simulink model "Full_model"  (R2020a)
settings: Solver=VariableStepAuto  StartTime=0.0  StopTime=inf  RelTol=1e-3
model workspace (MAT data in the model file):
  WinSize = Simulink.Parameter
  WinSize.Value = 16
  WinSize.DataType = 'double'
  WinSize.Dimensions = [1 1]
  fc_bandpass = Simulink.Parameter
  fc_bandpass.Value = [0.05 0.26]
  fc_bandpass.DataType = 'double'
  fc_bandpass.Dimensions = [1 2]
undefined symbols (not defined in the file or in its folder): A1, A30722, A91496, C1, currentCFG_Cognata_Amp_Tobi_split_UB, I1, J30722, P91496, UB, W1, W91496
libraries: gtecHighspeedLib x13, robotlib x6, dspnetwork x1, gUSBamplib x1, TobiiEyeTrackerLib x1
settings Model: Creator=LAB-OREN3  LastModifiedBy=LAB-OREN3

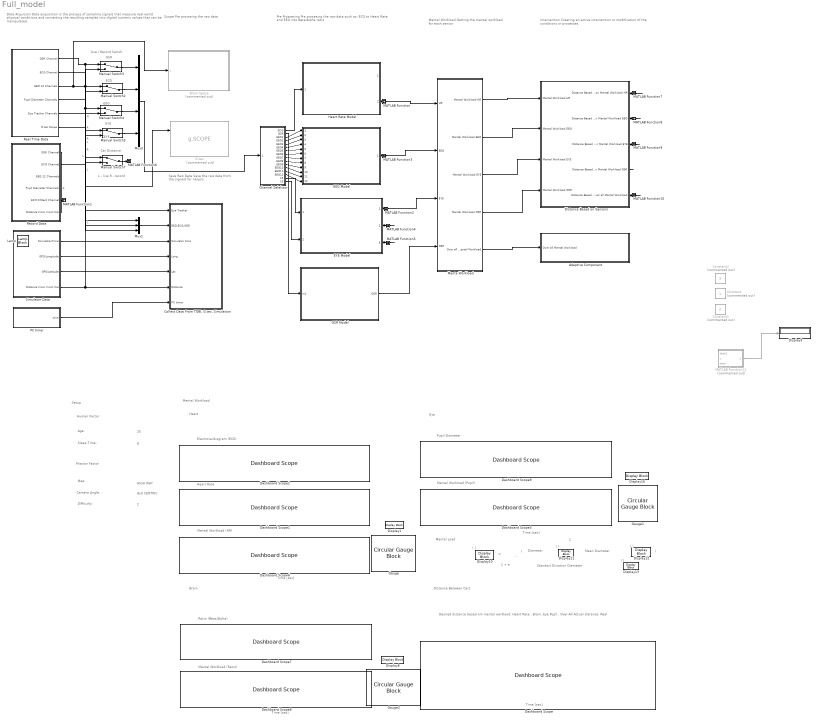
== system Full_model ==
  note: L - live
      | R - record
  note: Live / Record Switch
  note: GSR
  note: Intervention
      | Creating an active intervention or modification of the conditions or processes
  note: Save Raw Data
      | Save the raw data from the signals for nalysis
  note: Mental Workload
      | Getting the mental workload for each sensor
  note: Pre Prossesing
      | Pre prosseing the raw data such as:
      | ECG to Heart Rate and EEG into Beta/Alpha ratio
  note: Data Acquision
      | Data acquisition is the process of sampling signals that measure real-world physical conditions and converting the resulting samples into digital numeric values that can be manipulated.
  note: Time [sec]
  note: Electrocardiogram (ECG)
  note: . Distance Between Cars
  note: Mean Diameter
  note: 25
  note: Human Factor
  note: Standart Diviation Diameter
  note: Age:
  note: HIGH WAY
  note: Difficulty:
  note: Mental Workload (Pupil)
  note: ( )
  note: 8
  note: 1 + e
  note: Camera Angle: :
  note: Heart Rate
  note: Time [sec]
  note: Brain
  note: ( )
  note: Pupil Diameter
  note: . Setup
  note: 2
  note: ( )
  note: 1
  note: Desired distance based om mental worklaod:
      | Heart Rate , Brain, Eye Pupil , Over-All
      |
      | Actual distance: Real
  note: (
  note: Mission Factor
  note: Ratio (Beta/Alpha)
  note: -
  note: Mental Workload (HR)
  note: Sleep Time:
  note: ( )
  note: Diameter
  note: Mental Load
  note: )
  note: =
  note: Time [sec]
  note: Eye
  note: Mental Workload (Ratio)
  note: Time [sec]
  note: Mental Workload
  note: Heart
  note: Map:
  note: ALO CENTRIC
  note: ECG
  note: EEG
  note: EYE
  note: Car Distance
  note: EYE
  note: Scope
      | Pre prosseing the raw data
  Adaptive Component : Subsystem
  Brain Space : Subsystem  Commented=on
  Channel Selelctor : Subsystem
  "Collect Data From TOBI, G.tec, Simulation" : Subsystem
  Constant : Constant  Commented=on  SampleTime=0.5
  Constant1 : Constant  Commented=on  Value=2  SampleTime=0.5
  Constant2 : Constant  Commented=on  Value=3  SampleTime=0.5
  Dashboard Scope : DashboardScope  ShowInitialText=off  TimeSpan=10  Ymin=-1  Ymax=20  LegendPosition=Hide  ScaleAtStop=off
  Dashboard Scope1 : DashboardScope  TimeSpan=10  Ymin=0  Ymax=100  LegendPosition=Hide  ScaleAtStop=off
  Dashboard Scope2 : DashboardScope  TimeSpan=10  Ymin=-3000  Ymax=1000  LegendPosition=Hide  ScaleAtStop=off
  Dashboard Scope3 : DashboardScope  TimeSpan=10  Ymin=0  Ymax=1  LegendPosition=Hide  ScaleAtStop=off
  Dashboard Scope6 : DashboardScope  TimeSpan=10  Ymin=0  Ymax=1  LegendPosition=Hide  ScaleAtStop=off
  Dashboard Scope7 : DashboardScope  TimeSpan=10  Ymin=0  Ymax=0.5  LegendPosition=Hide  ScaleAtStop=off
  Dashboard Scope8 : DashboardScope  TimeSpan=10  Ymin=0  Ymax=1  LegendPosition=Hide  ScaleAtStop=off
  Dashboard Scope9 : DashboardScope  TimeSpan=10  Ymin=0  Ymax=5  LegendPosition=Hide  ScaleAtStop=off
  Display{1,8,10..11,13,16} (6 alike) : DisplayBlock  LabelPosition=Hide  Format=bank  Transparency=1
  Display12 : DisplayBlock  LabelPosition=Hide  Format=bank  Transparency=1  Layout=Fill available space
  Display3 : Display
  Distance Based on Sensors : Subsystem
  EEG Model : Subsystem  ReferencedSubsystem=EEG_Ratio_Model
  EYE Model : Subsystem  ReferencedSubsystem=Pupil_Diameter_Model
  G.tec : gtecHighspeedLib/g.SCOPE  Commented=on
      settings: SourceProductName=g.HIsys Library
  GSR Model : Subsystem
  Gauge : CircularGaugeBlock  LabelPosition=Hide  ScaleMax=1  TickInterval=0.2
  Gauge1 : CircularGaugeBlock  LabelPosition=Hide  ScaleMax=1  TickInterval=0.2
  Gauge2 : CircularGaugeBlock  LabelPosition=Hide  ScaleMax=1  TickInterval=0.2
  Heart Rate Model : Subsystem  ReferencedSubsystem=Heart_Rate_Model
  Lamp : LampBlock  LabelPosition=Hide
  MATLAB Function : MATLAB Function  TreatAsAtomicUnit=on
  MATLAB Function1 : MATLAB Function  TreatAsAtomicUnit=on
  MATLAB Function10 : MATLAB Function  TreatAsAtomicUnit=on
  MATLAB Function11 : MATLAB Function  Commented=on  TreatAsAtomicUnit=on
  MATLAB Function2 : MATLAB Function  TreatAsAtomicUnit=on
  MATLAB Function3 : MATLAB Function  TreatAsAtomicUnit=on
  MATLAB Function4 : MATLAB Function  TreatAsAtomicUnit=on
  MATLAB Function5 : MATLAB Function  TreatAsAtomicUnit=on
  MATLAB Function6 : MATLAB Function  TreatAsAtomicUnit=on
  MATLAB Function7 : MATLAB Function  TreatAsAtomicUnit=on
  MATLAB Function8 : MATLAB Function  TreatAsAtomicUnit=on
  MATLAB Function9 : MATLAB Function  TreatAsAtomicUnit=on
  Manual Switch{2..5,7} (5 alike) : ManualSwitch
  "Menta Workload " : Subsystem
  Mux1 : Mux  Inputs=3
  Mux3 : Mux
  PC timer : Subsystem
  Real Time Data : Subsystem
  Record Data : Subsystem
  Simulator Data : Subsystem
  wires:
  Simulator Data/2(GPS/Longitude) -> "Collect Data From TOBI, G.tec, Simulation"/4(Long)
  Simulator Data/3(GPS/Latitude) -> "Collect Data From TOBI, G.tec, Simulation"/5(Lat)
  Simulator Data/1(SimulationTime) -> "Collect Data From TOBI, G.tec, Simulation"/3(Simulator time)
  Simulator Data/4(Distance From Front Car) -> Manual Switch7/1, "Collect Data From TOBI, G.tec, Simulation"/6(Distance)  "L"
  Heart Rate Model/2 -> MATLAB Function/1(u)
  EYE Model/1 -> MATLAB Function2/1(u)
  GSR Model/1(GSR) -> "Menta Workload "/4(GSR)
  "Menta Workload "/2(Mental Workload EEG) -> Distance Based on Sensors/2(Mental Workload EEG)
  "Menta Workload "/5("Over all Mental Workload ") -> Adaptive Component/1("Over all Mental Workload ")
  Distance Based on Sensors/1(Distance Based on Mental Workload HR) -> MATLAB Function7/1(u)
  Distance Based on Sensors/2(Distance Based on Mental Workload EEG) -> MATLAB Function8/1(u)
  Distance Based on Sensors/3(Distance Based on Mental Workload EYE) -> MATLAB Function9/1(u)
  Distance Based on Sensors/4(Distance Based on Mental Workload GSR) -> ?
  Distance Based on Sensors/5(Distance Based on Over all Mental Workload) -> MATLAB Function10/1(u)
  EYE Model/2 -> MATLAB Function4/1(u)
  EYE Model/3 -> MATLAB Function5/1(u)
  Channel Selelctor/2(GSR) -> GSR Model/1(In1)
  Channel Selelctor/1(ECG) -> Heart Rate Model/1
  Channel Selelctor/3(EEG1) -> EEG Model/1
  Channel Selelctor/4(EEG2) -> EEG Model/2
  Channel Selelctor/5(EEG3) -> EEG Model/3
  Channel Selelctor/6(EEG4) -> EEG Model/4
  Channel Selelctor/7(EEG5) -> EEG Model/5
  Channel Selelctor/8(EEG6) -> EEG Model/6
  Channel Selelctor/9(EEG7) -> EEG Model/7
  Channel Selelctor/10(EEG8) -> EEG Model/8
  Channel Selelctor/11(EEG9) -> EEG Model/9
  Channel Selelctor/12(EEG10) -> EEG Model/10
  Channel Selelctor/13(EEG11) -> EEG Model/11
  Channel Selelctor/14(EEG12) -> EEG Model/12
  Channel Selelctor/15(Pupil right) -> EYE Model/1
  Channel Selelctor/16(Pupil Left) -> EYE Model/2
  Manual Switch3/1 -> Mux3/1
  Manual Switch2/1 -> Mux3/2
  Manual Switch4/1 -> Mux3/3
  Manual Switch5/1 -> Mux3/4
  Record Data/1(GSR Channel) -> Manual Switch3/2  "R"
  Real Time Data/1(GSR Channel) -> Manual Switch3/1, Mux1/1  "L"
  Real Time Data/2(ECG Channel) -> Mux1/2, Manual Switch2/1  "L"
  Record Data/2(ECG Channel) -> Manual Switch2/2  "R"
  Record Data/3(EEG 12 Channels) -> Manual Switch4/2  "R"
  Real Time Data/3(EEG 12 Channels) -> Mux1/3, Manual Switch4/1, Brain Space/1(L)  "L"
  Record Data/4(" Pupil Diameter Channels ") -> Manual Switch5/2  "R"
  Manual Switch7/1 -> MATLAB Function6/1(u)
  Record Data/5(ECG Filtterd Channel) -> MATLAB Function1/1(u)
  Real Time Data/5(Eye Tracker Channels) -> "Collect Data From TOBI, G.tec, Simulation"/1(Eye Tracker)
  Mux3/1 -> Channel Selelctor/1(16x1 vec)
  Mux1/1 -> "Collect Data From TOBI, G.tec, Simulation"/2("EEG,ECG,GSR ")
  Record Data/6(Distance From Front Car) -> Manual Switch7/2  "R"
  PC timer/1(time) -> "Collect Data From TOBI, G.tec, Simulation"/7(PC timer)
  Real Time Data/4(Pupil Diameter Channels) -> Manual Switch5/1
  MATLAB Function/1(y) -> "Menta Workload "/1(HR)
  MATLAB Function2/1(y) -> "Menta Workload "/3(EYE)
  EEG Model/1 -> MATLAB Function3/1(u)
  MATLAB Function3/1(y) -> "Menta Workload "/2(EEG)
  MATLAB Function4/1(y) -> ?
  MATLAB Function5/1(y) -> ?
  MATLAB Function7/1(y) -> ?
  MATLAB Function8/1(y) -> ?
  MATLAB Function9/1(y) -> ?
  MATLAB Function10/1(y) -> ?
  "Menta Workload "/3(Mental Workload EYE) -> Distance Based on Sensors/3(Mental Workload EYE)
  MATLAB Function11/1(y) -> Display3/1
  "Menta Workload "/1(Mental Workload HR) -> Distance Based on Sensors/1(Mental Workload HR)
  "Menta Workload "/4(Mental Workload GSR) -> Distance Based on Sensors/4(Mental Workload GSR)
  Real Time Data/6(G.tec Scope) -> G.tec/1

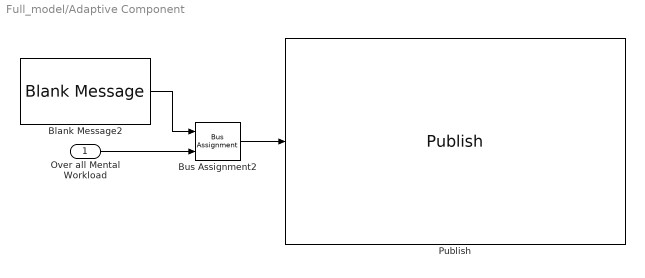
== system Full_model/Adaptive Component ==
  "Over all Mental Workload " : Inport
  Blank Message2 : robotlib/Blank Message  messageClass=Message  entityType=std_msgs/Float64  messageType=std_msgs/Float64  SampleTime=0
  Bus Assignment2 : BusAssignment  AssignedSignals=Data
  Publish : robotlib/Publish  topicSource=Specify your own  topic=/HR  messageType=std_msgs/Float64  messageQueueLength=1
  wires:
  "Over all Mental Workload "/1 -> Bus Assignment2/2
  Blank Message2/1 -> Bus Assignment2/1
  Bus Assignment2/1 -> Publish/1

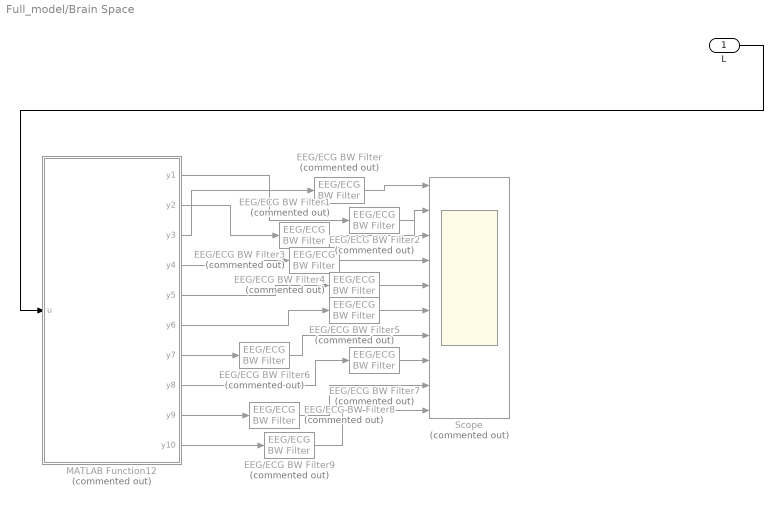
== system Full_model/Brain Space ==
  L : Inport
  EEG/ECG BW Filter{,1..9} (10 alike) : gtecHighspeedLib/EEG//ECG BW Filter  Commented=on  Order=6  LowerFreq=0.1  UpperFreq=30  SampFreq=512
      settings: SourceProductName=g.HIsys Library
  MATLAB Function12 : MATLAB Function  Commented=on  TreatAsAtomicUnit=on
  Scope : Scope  Commented=on  NumInputPorts=10
  wires:
  MATLAB Function12/1(y1) -> EEG/ECG BW Filter2/1
  MATLAB Function12/10(y10) -> EEG/ECG BW Filter9/1
  MATLAB Function12/4(y4) -> EEG/ECG BW Filter3/1
  MATLAB Function12/6(y6) -> EEG/ECG BW Filter5/1
  EEG/ECG BW Filter8/1 -> Scope/9
  EEG/ECG BW Filter3/1 -> Scope/4
  MATLAB Function12/2(y2) -> EEG/ECG BW Filter1/1
  EEG/ECG BW Filter5/1 -> Scope/6
  EEG/ECG BW Filter4/1 -> Scope/5
  EEG/ECG BW Filter7/1 -> Scope/8
  EEG/ECG BW Filter/1 -> Scope/1
  L/1 -> MATLAB Function12/1(u)
  MATLAB Function12/7(y7) -> EEG/ECG BW Filter6/1
  MATLAB Function12/8(y8) -> EEG/ECG BW Filter7/1
  EEG/ECG BW Filter1/1 -> Scope/2
  MATLAB Function12/9(y9) -> EEG/ECG BW Filter8/1
  MATLAB Function12/5(y5) -> EEG/ECG BW Filter4/1
  EEG/ECG BW Filter9/1 -> Scope/10
  EEG/ECG BW Filter2/1 -> Scope/3
  EEG/ECG BW Filter6/1 -> Scope/7
  MATLAB Function12/3(y3) -> EEG/ECG BW Filter/1

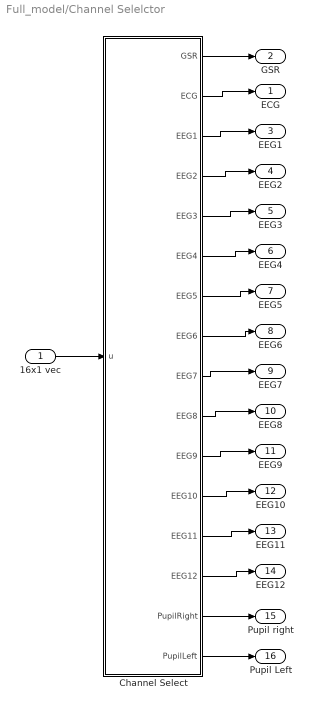
== system Full_model/Channel Selelctor ==
  16x1 vec : Inport
  " Channel Select" : MATLAB Function  TreatAsAtomicUnit=on
  ECG : Outport
  GSR : Outport  Port=2
  EEG1 : Outport  Port=3
  EEG2 : Outport  Port=4
  EEG3 : Outport  Port=5
  EEG4 : Outport  Port=6
  EEG5 : Outport  Port=7
  EEG6 : Outport  Port=8
  EEG7 : Outport  Port=9
  EEG8 : Outport  Port=10
  EEG9 : Outport  Port=11
  EEG10 : Outport  Port=12
  EEG11 : Outport  Port=13
  EEG12 : Outport  Port=14
  Pupil right : Outport  Port=15
  Pupil Left : Outport  Port=16
  wires:
  16x1 vec/1 -> " Channel Select"/1(u)
  " Channel Select"/1(GSR) -> GSR/1
  " Channel Select"/2(ECG) -> ECG/1
  " Channel Select"/3(EEG1) -> EEG1/1
  " Channel Select"/4(EEG2) -> EEG2/1
  " Channel Select"/5(EEG3) -> EEG3/1
  " Channel Select"/6(EEG4) -> EEG4/1
  " Channel Select"/7(EEG5) -> EEG5/1
  " Channel Select"/8(EEG6) -> EEG6/1
  " Channel Select"/9(EEG7) -> EEG7/1
  " Channel Select"/10(EEG8) -> EEG8/1
  " Channel Select"/11(EEG9) -> EEG9/1
  " Channel Select"/12(EEG10) -> EEG10/1
  " Channel Select"/13(EEG11) -> EEG11/1
  " Channel Select"/14(EEG12) -> EEG12/1
  " Channel Select"/15(PupilRight) -> Pupil right/1
  " Channel Select"/16(PupilLeft) -> Pupil Left/1

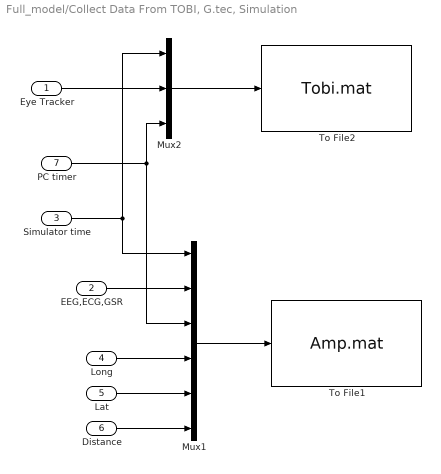
== system Full_model/Collect Data From TOBI, G.tec, Simulation ==
  Eye Tracker : Inport
  "EEG,ECG,GSR " : Inport  Port=2
  Simulator time : Inport  Port=3
  Long : Inport  Port=4
  Lat : Inport  Port=5
  Distance : Inport  Port=6
  PC timer : Inport  Port=7
  Mux1 : Mux  Inputs=6
  Mux2 : Mux  Inputs=3
  To File1 : ToFile  Filename=Amp.mat  MatrixName=Ampdata
  To File2 : ToFile  Filename=Tobi.mat  MatrixName=Tobidata
  wires:
  Eye Tracker/1 -> Mux2/2
  Simulator time/1 -> Mux1/1, Mux2/1
  Mux1/1 -> To File1/1
  Mux2/1 -> To File2/1
  Long/1 -> Mux1/4
  Distance/1 -> Mux1/6
  "EEG,ECG,GSR "/1 -> Mux1/2
  Lat/1 -> Mux1/5
  PC timer/1 -> Mux1/3, Mux2/3

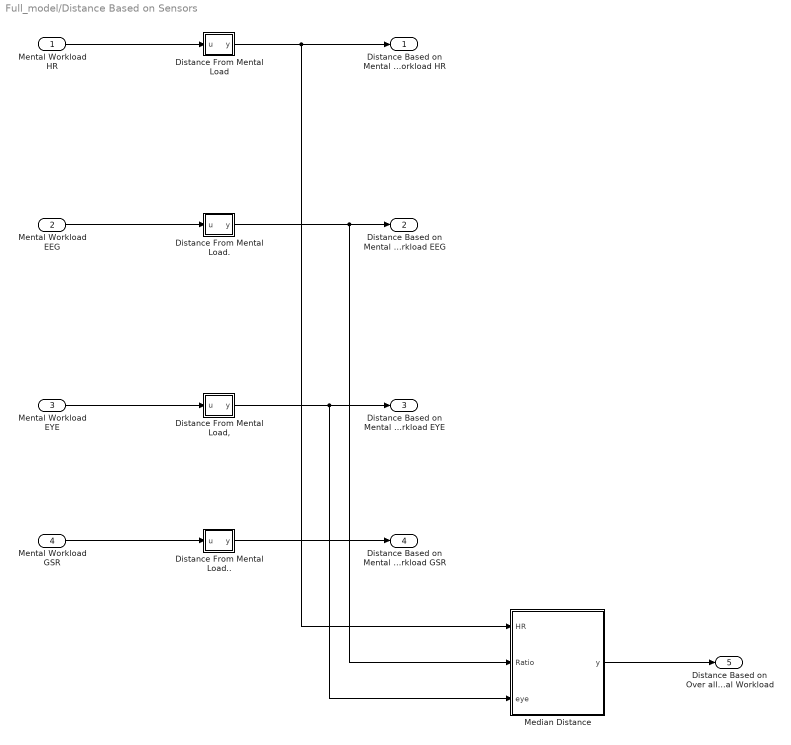
== system Full_model/Distance Based on Sensors ==
  Mental Workload HR : Inport
  Mental Workload EEG : Inport  Port=2
  Mental Workload EYE : Inport  Port=3
  Mental Workload GSR : Inport  Port=4
  Distance From Mental Load : MATLAB Function  TreatAsAtomicUnit=on
  Distance From Mental Load, : MATLAB Function  TreatAsAtomicUnit=on
  Distance From Mental Load. : MATLAB Function  TreatAsAtomicUnit=on
  Distance From Mental Load.. : MATLAB Function  TreatAsAtomicUnit=on
  Median Distance : MATLAB Function  TreatAsAtomicUnit=on
  Distance Based on Mental Workload HR : Outport
  Distance Based on Mental Workload EEG : Outport  Port=2
  Distance Based on Mental Workload EYE : Outport  Port=3
  Distance Based on Mental Workload GSR : Outport  Port=4
  Distance Based on Over all Mental Workload : Outport  Port=5
  wires:
  Distance From Mental Load,/1(y) -> Distance Based on Mental Workload EYE/1, Median Distance/3(eye)
  Mental Workload HR/1 -> Distance From Mental Load/1(u)
  Distance From Mental Load../1(y) -> Distance Based on Mental Workload GSR/1
  Mental Workload EEG/1 -> Distance From Mental Load./1(u)
  Mental Workload GSR/1 -> Distance From Mental Load../1(u)
  Distance From Mental Load/1(y) -> Distance Based on Mental Workload HR/1, Median Distance/1(HR)
  Mental Workload EYE/1 -> Distance From Mental Load,/1(u)
  Distance From Mental Load./1(y) -> Distance Based on Mental Workload EEG/1, Median Distance/2(Ratio)
  Median Distance/1(y) -> Distance Based on Over all Mental Workload/1

== system Full_model/GSR Model ==
  In1 : Inport
  GSR : Outport
  wires:
  In1/1 -> GSR/1

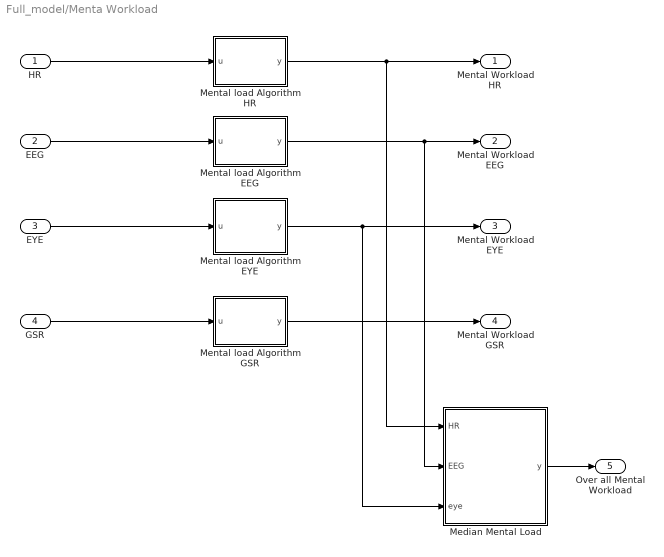
== system Full_model/Menta Workload  ==
  HR : Inport
  EEG : Inport  Port=2
  EYE : Inport  Port=3
  GSR : Inport  Port=4
  Median Mental Load : MATLAB Function  TreatAsAtomicUnit=on
  Mental load Algorithm EEG : MATLAB Function  TreatAsAtomicUnit=on
  Mental load Algorithm EYE : MATLAB Function  TreatAsAtomicUnit=on
  Mental load Algorithm GSR : MATLAB Function  TreatAsAtomicUnit=on
  Mental load Algorithm HR : MATLAB Function  TreatAsAtomicUnit=on
  Mental Workload HR : Outport
  Mental Workload EEG : Outport  Port=2
  Mental Workload EYE : Outport  Port=3
  Mental Workload GSR : Outport  Port=4
  "Over all Mental Workload " : Outport  Port=5
  wires:
  HR/1 -> Mental load Algorithm HR/1(u)
  Mental load Algorithm HR/1(y) -> Mental Workload HR/1, Median Mental Load/1(HR)
  EEG/1 -> Mental load Algorithm EEG/1(u)
  Mental load Algorithm EEG/1(y) -> Median Mental Load/2(EEG), Mental Workload EEG/1
  EYE/1 -> Mental load Algorithm EYE/1(u)
  Mental load Algorithm EYE/1(y) -> Mental Workload EYE/1, Median Mental Load/3(eye)
  GSR/1 -> Mental load Algorithm GSR/1(u)
  Mental load Algorithm GSR/1(y) -> Mental Workload GSR/1
  Median Mental Load/1(y) -> "Over all Mental Workload "/1

== system Full_model/PC timer ==
  PC timer : MATLAB Function  TreatAsAtomicUnit=on
  time : Outport
  wires:
  PC timer/1(z) -> time/1

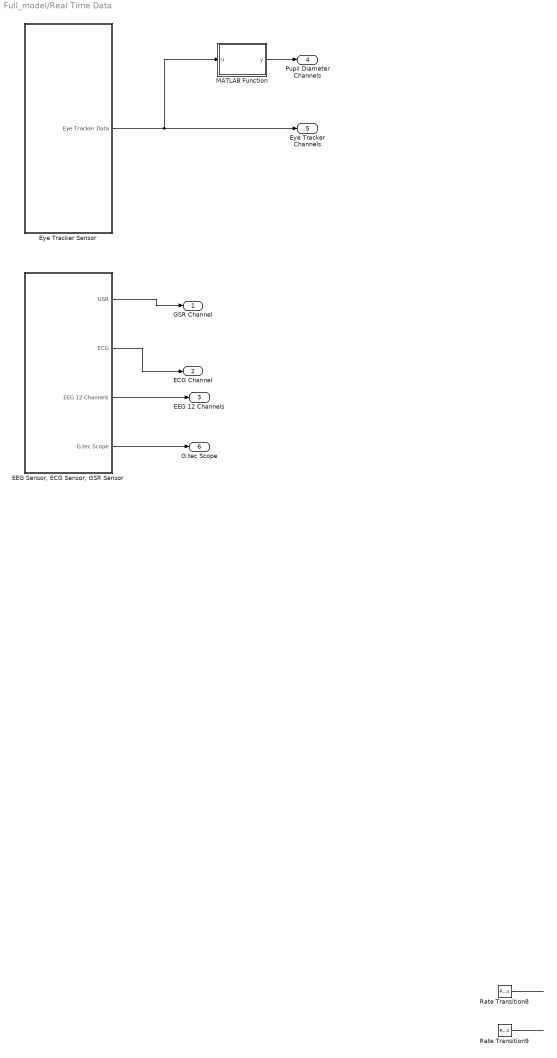
== system Full_model/Real Time Data ==
  "EEG Sensor, ECG Sensor, GSR Sensor " : Subsystem
  Eye Tracker Sensor : Subsystem
  MATLAB Function : MATLAB Function  TreatAsAtomicUnit=on
  Rate Transition8 : RateTransition  Deterministic=off  OutPortSampleTimeOpt=Inherit
  Rate Transition9 : RateTransition  Deterministic=off  OutPortSampleTimeOpt=Inherit
  GSR Channel : Outport
  ECG Channel : Outport  Port=2
  EEG 12 Channels : Outport  Port=3
  Pupil Diameter Channels : Outport  Port=4
  Eye Tracker Channels : Outport  Port=5
  G.tec Scope : Outport  Port=6
  wires:
  Eye Tracker Sensor/1(Eye Tracker Data) -> MATLAB Function/1(u), Eye Tracker Channels/1
  Rate Transition8/1 -> ?
  Rate Transition9/1 -> ?
  "EEG Sensor, ECG Sensor, GSR Sensor "/1(GSR) -> GSR Channel/1
  "EEG Sensor, ECG Sensor, GSR Sensor "/2(ECG) -> ECG Channel/1
  "EEG Sensor, ECG Sensor, GSR Sensor "/3(EEG 12 Channels) -> EEG 12 Channels/1
  MATLAB Function/1(y) -> Pupil Diameter Channels/1
  "EEG Sensor, ECG Sensor, GSR Sensor "/4(G.tec Scope) -> G.tec Scope/1

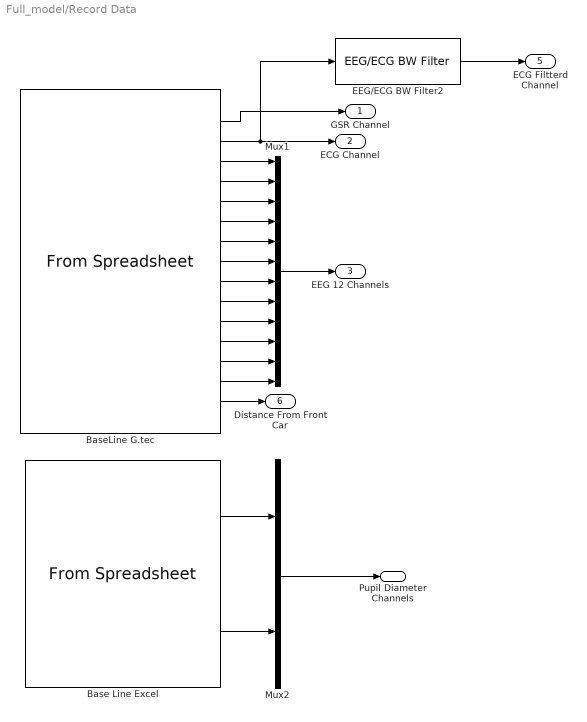
== system Full_model/Record Data ==
  Base Line Excel : FromSpreadsheet  FileName=C:\Users\LAB-OREN3\Desktop\CognataData\Participants_DATA\Test\3\Tobii Data of A3_458493_COMBINED_CAR_DELAY_50_TTC_15 at (18_15_7).xlsx  SheetName=גיליון1  Range=A1:A30722,I1:J30722  SampleTime=0.001953125
  BaseLine G.tec : FromSpreadsheet  FileName=C:\Users\LAB-OREN3\Desktop\CognataData\Participants_DATA\Test\1\g.techAmp Data of A6_473257_COMBINED_CUBE_DELAY_150_TTC_ML at (13;32;25).xlsx  SheetName=גיליון1  Range=A1:A91496,C1:P91496,W1:W91496  SampleTime=0.001953125
  EEG/ECG BW Filter2 : gtecHighspeedLib/EEG//ECG BW Filter  Order=6  LowerFreq=0.1  UpperFreq=30  SampFreq=512
      settings: SourceProductName=g.HIsys Library
  Mux1 : Mux  Inputs=12
  Mux2 : Mux  Inputs=2
  GSR Channel : Outport
  ECG Channel : Outport  Port=2
  EEG 12 Channels : Outport  Port=3
  " Pupil Diameter Channels " : Outport  Port=4
  ECG Filtterd Channel : Outport  Port=5
  Distance From Front Car : Outport  Port=6
  wires:
  BaseLine G.tec/5 -> Mux1/3
  BaseLine G.tec/13 -> Mux1/11
  BaseLine G.tec/10 -> Mux1/8
  BaseLine G.tec/11 -> Mux1/9
  BaseLine G.tec/14 -> Mux1/12
  BaseLine G.tec/12 -> Mux1/10
  BaseLine G.tec/8 -> Mux1/6
  BaseLine G.tec/4 -> Mux1/2
  BaseLine G.tec/9 -> Mux1/7
  BaseLine G.tec/6 -> Mux1/4
  BaseLine G.tec/7 -> Mux1/5
  BaseLine G.tec/3 -> Mux1/1
  BaseLine G.tec/15 -> Distance From Front Car/1
  BaseLine G.tec/2 -> ECG Channel/1, EEG/ECG BW Filter2/1
  BaseLine G.tec/1 -> GSR Channel/1
  Base Line Excel/2 -> Mux2/2
  Base Line Excel/1 -> Mux2/1
  Mux2/1 -> " Pupil Diameter Channels "/1
  EEG/ECG BW Filter2/1 -> ECG Filtterd Channel/1
  Mux1/1 -> EEG 12 Channels/1

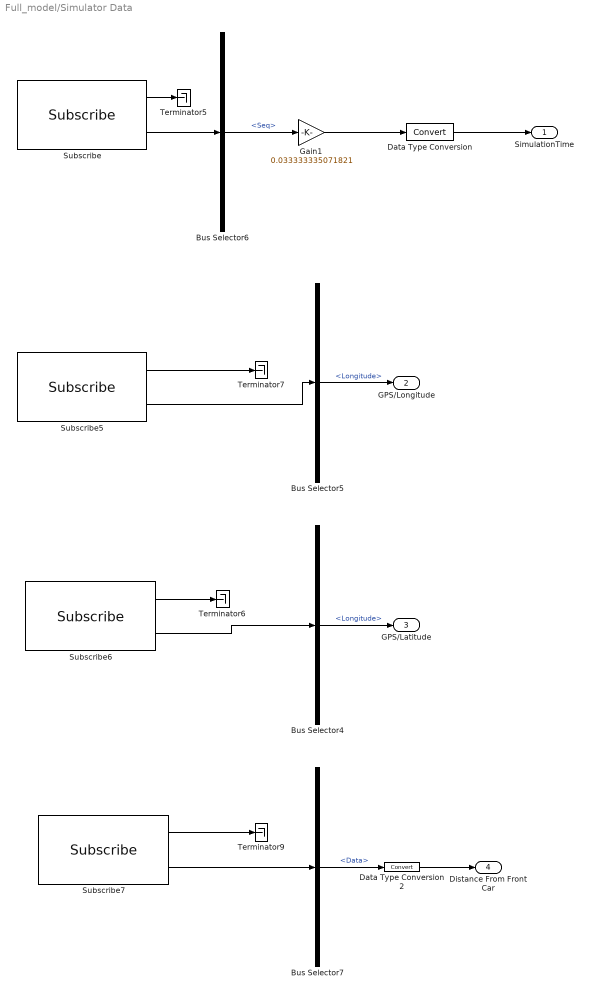
== system Full_model/Simulator Data ==
  Bus Selector4 : BusSelector  OutputSignals=Longitude
  Bus Selector5 : BusSelector  OutputSignals=Longitude
  Bus Selector6 : BusSelector  OutputSignals=Header.Seq
  Bus Selector7 : BusSelector  OutputSignals=Data
  Data Type Conversion : DataTypeConversion
  Data Type Conversion2 : DataTypeConversion
  Gain1 : Gain  Gain=0.033333335071821
  Subscribe : robotlib/Subscribe  topicSource=Specify your own  topic=/cognataSDK/GPS/info  messageType=sensor_msgs/NavSatFix  sampleTime=0.5  messageQueueLength=1
  Subscribe5 : robotlib/Subscribe  topicSource=Specify your own  topic=/cognataSDK/GPS/info  messageType=sensor_msgs/NavSatFix  sampleTime=-1  messageQueueLength=1
  Subscribe6 : robotlib/Subscribe  topicSource=Specify your own  topic=/cognataSDK/GPS/info  messageType=sensor_msgs/NavSatFix  sampleTime=-1  messageQueueLength=1
  Subscribe7 : robotlib/Subscribe  topicSource=Specify your own  topic=/Distance_topic  messageType=std_msgs/Float32  sampleTime=0.5  messageQueueLength=1
  Terminator{5..7,9} (4 alike) : Terminator
  SimulationTime : Outport
  GPS/Longitude : Outport  Port=2
  GPS/Latitude : Outport  Port=3
  Distance From Front Car : Outport  Port=4
  wires:
  Subscribe/1 -> Terminator5/1
  Bus Selector4/1 -> GPS/Latitude/1  "<Longitude>"
  Subscribe6/2 -> Bus Selector4/1
  Subscribe6/1 -> Terminator6/1
  Bus Selector5/1 -> GPS/Longitude/1  "<Longitude>"
  Subscribe5/2 -> Bus Selector5/1
  Subscribe5/1 -> Terminator7/1
  Subscribe/2 -> Bus Selector6/1
  Bus Selector6/1 -> Gain1/1  "<Seq>"
  Subscribe7/2 -> Bus Selector7/1
  Subscribe7/1 -> Terminator9/1
  Bus Selector7/1 -> Data Type Conversion2/1  "<Data>"
  Gain1/1 -> Data Type Conversion/1
  Data Type Conversion/1 -> SimulationTime/1
  Data Type Conversion2/1 -> Distance From Front Car/1

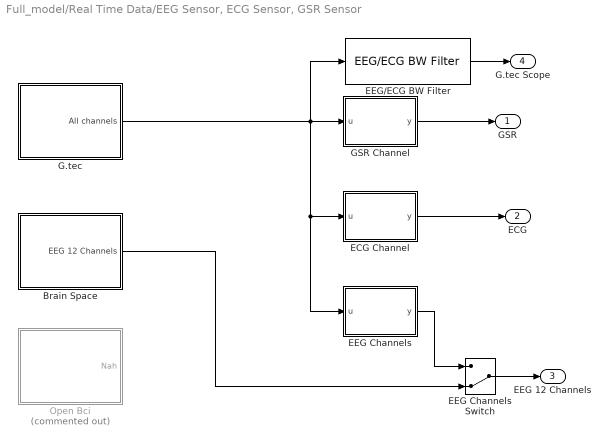
== system Full_model/Real Time Data/EEG Sensor, ECG Sensor, GSR Sensor  ==
  Brain Space : Subsystem
  "ECG Channel " : MATLAB Function  TreatAsAtomicUnit=on
  "EEG Channels " : MATLAB Function  TreatAsAtomicUnit=on
  EEG Channels Switch : ManualSwitch  CurrentSetting=0
  EEG/ECG BW Filter : gtecHighspeedLib/EEG//ECG BW Filter  Order=6  LowerFreq=0.1  UpperFreq=30  SampFreq=512
      settings: SourceProductName=g.HIsys Library
  G.tec : Subsystem
  GSR Channel : MATLAB Function  TreatAsAtomicUnit=on
  Open Bci : Subsystem  Commented=on
  GSR : Outport
  ECG : Outport  Port=2
  EEG 12 Channels : Outport  Port=3
  G.tec Scope : Outport  Port=4
  wires:
  G.tec/1(All channels) -> "EEG Channels "/1(u), "ECG Channel "/1(u), GSR Channel/1(u), EEG/ECG BW Filter/1
  GSR Channel/1(y) -> GSR/1
  "ECG Channel "/1(y) -> ECG/1
  "EEG Channels "/1(y) -> EEG Channels Switch/1
  Brain Space/1(EEG 12 Channels) -> EEG Channels Switch/2
  EEG Channels Switch/1 -> EEG 12 Channels/1
  EEG/ECG BW Filter/1 -> G.tec Scope/1

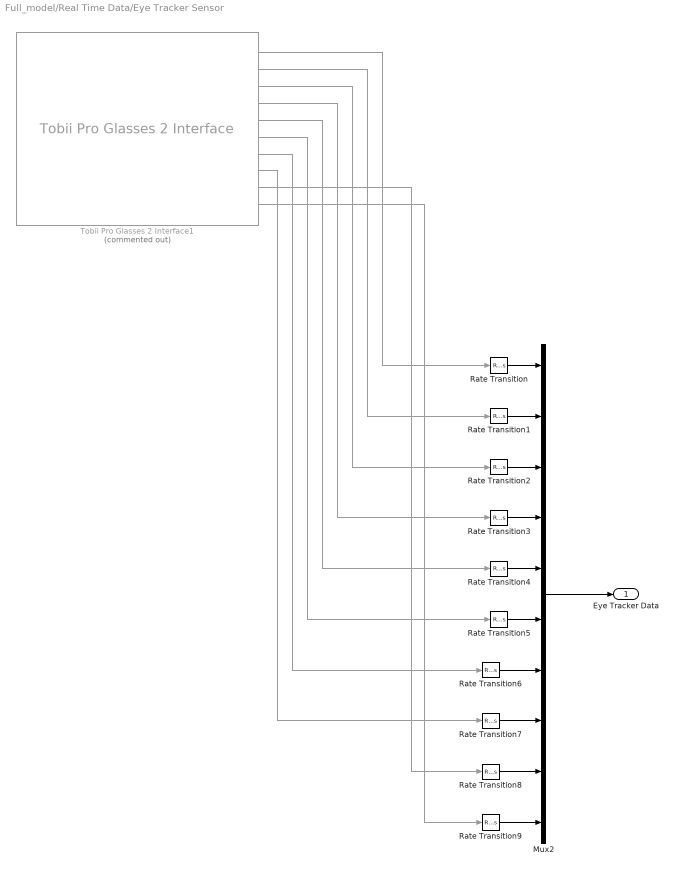
== system Full_model/Real Time Data/Eye Tracker Sensor ==
  Mux2 : Mux  Inputs=10
  Rate Transition{,1..9} (10 alike) : RateTransition  Deterministic=off  OutPortSampleTimeOpt=Inherit
  Tobii Pro Glasses 2 Interface1 : TobiiEyeTrackerLib/Tobii Pro Glasses 2 Interface  Commented=on  Key=0  pc_right=off  pc_left=off  pd_right=off  pd_left=off  gd_right=off  gd_left=off  gp=on  gp3=off  gy=off  ac=off
      settings: SourceProductName=g.EYEtracking Interface (Tobii Pro Glasses 2)
  Eye Tracker Data : Outport
  wires:
  Rate Transition2/1 -> Mux2/3
  Rate Transition6/1 -> Mux2/7
  Tobii Pro Glasses 2 Interface1/1 -> Rate Transition/1
  Rate Transition1/1 -> Mux2/2
  Mux2/1 -> Eye Tracker Data/1
  Tobii Pro Glasses 2 Interface1/8 -> Rate Transition7/1
  Tobii Pro Glasses 2 Interface1/5 -> Rate Transition4/1
  Tobii Pro Glasses 2 Interface1/10 -> Rate Transition9/1
  Tobii Pro Glasses 2 Interface1/2 -> Rate Transition1/1
  Tobii Pro Glasses 2 Interface1/9 -> Rate Transition8/1
  Tobii Pro Glasses 2 Interface1/7 -> Rate Transition6/1
  Rate Transition/1 -> Mux2/1
  Rate Transition4/1 -> Mux2/5
  Tobii Pro Glasses 2 Interface1/6 -> Rate Transition5/1
  Rate Transition5/1 -> Mux2/6
  Rate Transition3/1 -> Mux2/4
  Rate Transition8/1 -> Mux2/9
  Rate Transition9/1 -> Mux2/10
  Rate Transition7/1 -> Mux2/8
  Tobii Pro Glasses 2 Interface1/4 -> Rate Transition3/1
  Tobii Pro Glasses 2 Interface1/3 -> Rate Transition2/1

== system Full_model/Real Time Data/EEG Sensor, ECG Sensor, GSR Sensor /Brain Space ==
  Reshape : Reshape
  UDP Receive : dspnetwork/UDP Receive  localURL='0.0.0.0'  localPort=5005  remoteURL='0.0.0.0'  remotePort=-1  recvBufferSize=8192  dims=12  signalDatatype=double  isComplex=off  isVarSize=off  showBlockingTime=off  blockingTime=0  sampletime=0.001953125  blockPlatform=[]
  EEG 12 Channels : Outport
  wires:
  UDP Receive/1 -> Reshape/1
  UDP Receive/2 -> ?
  Reshape/1 -> EEG 12 Channels/1

== system Full_model/Real Time Data/EEG Sensor, ECG Sensor, GSR Sensor /G.tec ==
  G.tec : gUSBamplib/g.USBamp  cfg=currentCFG_Cognata_Amp_Tobi_split_UB-2015.09.13.cfg  snr=UB-2015.09.13
      settings: SourceProductName=g.USBamp
  Input Adaptation : Subsystem
  All channels : Outport
  wires:
  G.tec/1 -> Input Adaptation/1(In)
  Input Adaptation/1(All channels) -> All channels/1

== system Full_model/Real Time Data/EEG Sensor, ECG Sensor, GSR Sensor /Open Bci ==
  Nah : Outport
  wires:
  ? -> Nah/1

== system Full_model/Real Time Data/EEG Sensor, ECG Sensor, GSR Sensor /G.tec/Input Adaptation ==
  In : Inport
  Data Type Conversion : DataTypeConversion  OutDataTypeStr=double
  Unbuffer : Unbuffer
  All channels : Outport
  wires:
  In/1 -> Unbuffer/1
  Unbuffer/1 -> Data Type Conversion/1
  Data Type Conversion/1 -> All channels/1

== matlab function Full_model/Distance Based on Sensors/Distance From Mental Load. ==
  data: u input; y output
function y = fcn(u)
%#codegen

y = (u*10)+10;

== matlab function Full_model/Real Time Data/EEG Sensor, ECG Sensor, GSR Sensor /EEG Channels  ==
  data: u input; y output
function y = fcn(u)

y = u(3:14);

== matlab function Full_model/MATLAB Function2 ==
  data: u input; y output
function y = fcn(u)

y = u;

== matlab function Full_model/Channel Selelctor/ Channel Select ==
  data: GSR output; u input; ECG output; EEG1 output; EEG2 output; EEG3 output; EEG4 output; EEG5 output; EEG6 output; EEG7 output; EEG8 output; EEG9 output; EEG10 output; EEG11 output; EEG12 output; PupilRight output; PupilLeft output
function [GSR, ECG, EEG1, EEG2, EEG3, EEG4, EEG5, EEG6, EEG7, EEG8, EEG9, EEG10, EEG11, EEG12, PupilRight, PupilLeft] = fcn(u)

GSR = u(1);
ECG = u(2);
EEG1 = u(3);
EEG2 = u(4);
EEG3 = u(5);
EEG4 = u(6);
EEG5 = u(7);
EEG6 = u(8);
EEG7 = u(9);
EEG8 = u(10);
EEG9 = u(11);
EEG10 = u(12);
EEG11 = u(13);
EEG12 = u(14);
PupilRight = u(15);
PupilLeft = u(16);

== matlab function Full_model/MATLAB Function3 ==
  data: u input; y output
function y = fcn(u)

y = u;

== matlab function Full_model/MATLAB Function4 ==
  data: u input; y output
function y = fcn(u)

y = u;

== matlab function Full_model/MATLAB Function5 ==
  data: u input; y output
function y = fcn(u)

y = u;

== matlab function Full_model/MATLAB Function6 ==
  data: u input; y output
function y = fcn(u)

y = u;

== matlab function Full_model/MATLAB Function7 ==
  data: u input; y output
function y = fcn(u)

y = u;

== matlab function Full_model/MATLAB Function8 ==
  data: u input; y output
function y = fcn(u)

y = u;

== matlab function Full_model/MATLAB Function9 ==
  data: u input; y output
function y = fcn(u)

y = u;

== matlab function Full_model/MATLAB Function10 ==
  data: u input; y output
function y = fcn(u)

y = u;

== matlab function Full_model/MATLAB Function11 ==
  data: data1 input; u input; y output; data input
function y = fcn(data1, u, data)


y= test_for_py(u, data, data1);

end

== matlab function Full_model/Brain Space/MATLAB Function12 ==
  data: u input; y1 output; y2 output; y3 output; y4 output; y5 output; y6 output; y7 output; y8 output; y9 output; y10 output
function [y1,y2,y3,y4,y5,y6,y7,y8,y9,y10] = fcn(u)

y1 = u(1);
y2 = u(2);
y3 = u(3);
y4 = u(4);
y5 = u(5);
y6 = u(6);
y7 = u(7);
y8 = u(8);
y9 = u(9);
y10 = u(10);

== matlab function Full_model/Distance Based on Sensors/Distance From Mental Load ==
  data: u input; y output
function y = fcn(u)
%#codegen

y = (u*10)+10;

== matlab function Full_model/Menta Workload /Mental load Algorithm EYE ==
  data: u input; y output
function y = fcn( u)

y= probability_of_metal_load_EYE(u);

end

== matlab function Full_model/Distance Based on Sensors/Distance From Mental Load.. ==
  data: u input; y output
function y = fcn(u)
%#codegen

y = (u*10)+10;

== matlab function Full_model/Menta Workload /Mental load Algorithm GSR ==
  data: u input; y output
function y = fcn(u)

y= probability_of_metal_load_GSR(u);

end

== matlab function Full_model/Distance Based on Sensors/Distance From Mental Load, ==
  data: u input; y output
function y = fcn(u)
%#codegen

y = (u*10)+10;

== matlab function Full_model/Real Time Data/MATLAB Function ==
  data: u input; y output
function y = fcn(u)

y = u(3:4);

== matlab function Full_model/MATLAB Function ==
  data: u input; y output
function y = fcn(u)

y = u;

== matlab function Full_model/MATLAB Function1 ==
  data: u input; y output
function y = fcn(u)

y = u;

== matlab function Full_model/Menta Workload /Mental load Algorithm HR ==
  data: u input; y output
function y = fcn(u)

y= probability_of_mental_load_HR(u);

end

== matlab function Full_model/Distance Based on Sensors/Median Distance ==
  data: HR input; y output; Ratio input; eye input
function y = fcn(HR, Ratio, eye)


    vac = [HR,Ratio,eye];
    y = median(vac);

end

== matlab function Full_model/Menta Workload /Mental load Algorithm EEG ==
  data: u input; y output
function y = fcn(u)

y= probability_of_metal_load_EEG(u);

end

== matlab function Full_model/PC timer/PC timer ==
  data: z output
function z = fcn()
eml.extrinsic('clock'); 
t = [0,0,0,0,0,0];
t = clock;
k = t(1,4:6);
z = k';
end

== matlab function Full_model/Real Time Data/EEG Sensor, ECG Sensor, GSR Sensor /GSR Channel ==
  data: u input; y output
function y = fcn(u)

y = u(1);

== matlab function Full_model/Menta Workload /Median Mental Load ==
  data: HR input; y output; EEG input; eye input
function y = fcn(HR, EEG, eye)


    vac = [HR, EEG, eye];
    y = median(vac);

end

== matlab function Full_model/Real Time Data/EEG Sensor, ECG Sensor, GSR Sensor /ECG Channel  ==
  data: u input; y output
function y = fcn(u)

y = u(2);
